simulink model "test_trajectories_num"  (Simulink 7.7)
settings: Solver=ode45  StartTime=0.0  StopTime=2  MaxStep=Step_Time  RelTol=1e-3
values from neighbouring files (symbols this model uses):
  q0 = homeConfiguration(robot)    [inv_example.m]
settings Model: Creator=saeed  LastModifiedBy=Other
settings CodeAppCC: CustomSymbolStrType=$N$R$M_T
settings GRTTargetCC: TargetFunctionLibrary=NOT IN USE  CPPClassGenCompliant=on

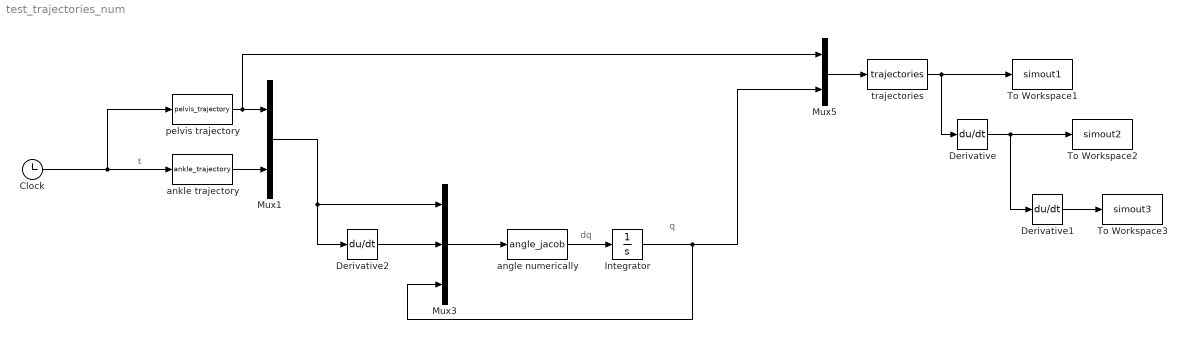
== system test_trajectories_num ==
  note: dq
  note: q
  Clock : Clock
      settings: Decimation=10
  Derivative : Derivative
  Derivative1 : Derivative
  Derivative2 : Derivative
  Integrator : Integrator  InitialCondition=q0
  Mux1 : Mux  Inputs=2
  Mux3 : Mux  Inputs=3
  Mux5 : Mux  Inputs=2
  To Workspace1 : ToWorkspace  VariableName=simout1  SampleTime=-1  SaveFormat=Structure With Time
  To Workspace2 : ToWorkspace  VariableName=simout2  SampleTime=-1  SaveFormat=Structure With Time
  To Workspace3 : ToWorkspace  VariableName=simout3  SampleTime=-1  SaveFormat=Structure With Time
  angle numerically : MATLABFcn  MATLABFcn=angle_jacob
  ankle trajectory : MATLABFcn  MATLABFcn=ankle_trajectory
  pelvis trajectory : MATLABFcn  MATLABFcn=pelvis_trajectory
  trajectories : MATLABFcn  MATLABFcn=trajectories
  wires:
  Clock/1 -> ankle trajectory/1, pelvis trajectory/1  "t"
  pelvis trajectory/1 -> Mux1/1, Mux5/1
  ankle trajectory/1 -> Mux1/2
  Mux5/1 -> trajectories/1
  trajectories/1 -> To Workspace1/1, Derivative/1
  Derivative/1 -> Derivative1/1, To Workspace2/1
  Derivative1/1 -> To Workspace3/1
  Derivative2/1 -> Mux3/2
  Mux3/1 -> angle numerically/1
  angle numerically/1 -> Integrator/1
  Integrator/1 -> Mux3/3, Mux5/2
  Mux1/1 -> Mux3/1, Derivative2/1
